simulink model "chap15_2sim"  (Simulink 8.1)
settings: Solver=ode45  StartTime=0.0  StopTime=10  FixedStep=0.005  RelTol=1e-3
settings Model: Creator=hp  LastModifiedBy=liujk  ExtModeTrigMode=oneshot  ExtModeArmWhenConnect=off
settings DataIOCC: LimitDataPoints=off  SignalLoggingName=sigsOut
settings OptimizationCC: BooleanDataType=off  InitFltsAndDblsToZero=on
settings DebuggingCC: SaveWithParameterizedLinksMsg=none  SignalResolutionControl=TryResolveAllWithWarning  SolverPrmCheckMsg=none  MultiTaskDSMMsg=warning  MultiTaskCondExecSysMsg=none  StrictBusMsg=None
settings HardwareCC: TargetUnknown=on
settings RTWCC: IncludeERTFirstTime=on
settings GRTTargetCC: TargetFcnLib=ansi_tfl_tmw.mat

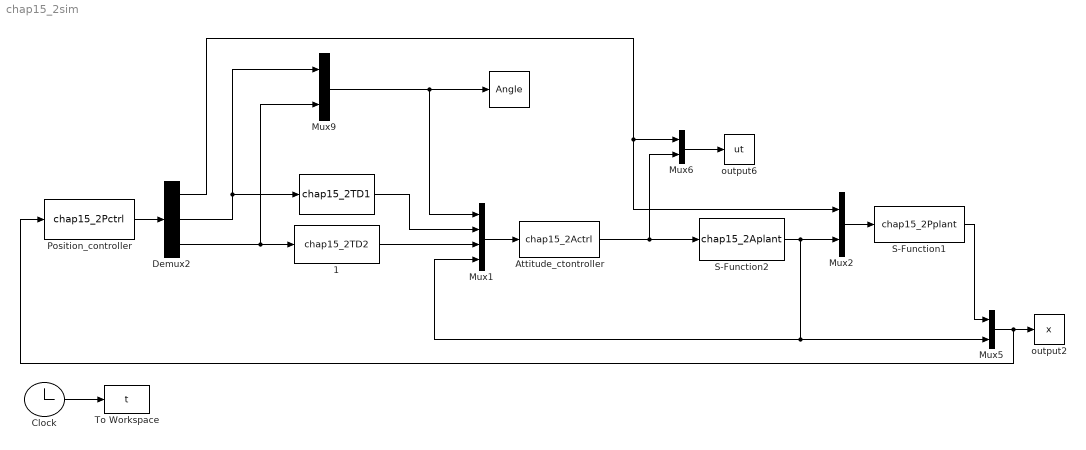
== system chap15_2sim ==
  " " : S-Function  FunctionName=chap15_2TD1  EnableBusSupport=off
  "   " : ToWorkspace  VariableName=Angle  SampleTime=-1
  " 1" : S-Function  FunctionName=chap15_2TD2  EnableBusSupport=off
  Attitude_ctontroller : S-Function  FunctionName=chap15_2Actrl  EnableBusSupport=off
  Clock : Clock
  Demux2 : Demux  Outputs=3
  Mux1 : Mux
  Mux{2,5..6,9} (4 alike) : Mux  Inputs=2
  Position_controller : S-Function  FunctionName=chap15_2Pctrl  EnableBusSupport=off
  S-Function1 : S-Function  FunctionName=chap15_2Pplant  EnableBusSupport=off
  S-Function2 : S-Function  FunctionName=chap15_2Aplant  EnableBusSupport=off
  To Workspace : ToWorkspace  VariableName=t  SampleTime=-1
  output2 : ToWorkspace  VariableName=x  SampleTime=-1
  output6 : ToWorkspace  VariableName=ut  SampleTime=-1
  wires:
  Clock/1 -> To Workspace/1
  Mux2/1 -> S-Function1/1
  S-Function2/1 -> Mux2/2, Mux5/2, Mux1/4
  Mux5/1 -> Position_controller/1, output2/1
  Demux2/2 -> Mux9/1, " "/1
  Demux2/1 -> Mux6/1, Mux2/1
  Demux2/3 -> Mux9/2, " 1"/1
  Mux1/1 -> Attitude_ctontroller/1
  Attitude_ctontroller/1 -> S-Function2/1, Mux6/2
  Position_controller/1 -> Demux2/1
  Mux6/1 -> output6/1
  Mux9/1 -> "   "/1, Mux1/1
  S-Function1/1 -> Mux5/1
  " "/1 -> Mux1/2
  " 1"/1 -> Mux1/3
